simulink model "slidemodecontrol2"  (R2017b)
settings: Solver=ode45  StartTime=0.0  StopTime=2500  FixedStep=0.01  MaxStep=0.04  RelTol=1e-3
values from neighbouring files (symbols this model uses):
  azi0 = 90/180*pi    (= 1.57079632679)    [MonteCarlo_f.m]    (also in MonteCarlo_l.m; MonteCarlo_s.m; calcu_delta.m = 0.174532925199; calcu_delta11.m)
  cd0 = 0.024    [flight_sim.m]
  cd1 = 7.24e-4    (= 0.000724)    [flight_sim.m]
  cd2 = 0.406    [flight_sim.m]
  cl0 = -0.2317    [flight_sim.m]
  cl1 = 0.0513    [flight_sim.m]
  cl2 = 0.2945    [flight_sim.m]
  delta_d = delta_d0(ii)    [MonteCarlo_f.m]    (also in MonteCarlo_l.m; MonteCarlo_s.m; calcu_delta11.m = -0.08; calcu_delta3.m = -0.079)
  delta_l = delta_l0(ii)    [MonteCarlo_f.m]    (also in MonteCarlo_l.m; MonteCarlo_s.m; calcu_delta3.m = 0.05)
  fpa0 = theta_0(ii)    [MonteCarlo_f.m]    (also in MonteCarlo_l.m; MonteCarlo_s.m; calcu_delta.m = -0.0349065850399; calcu_delta11.m = -0.0349065850399)
  hs = 7320    [constant.m]    (also in flight_sim.m)
  lat0 = 0    [MonteCarlo_f.m]    (also in MonteCarlo_l.m; MonteCarlo_s.m; calcu_delta.m; calcu_delta11.m)
  lon0 = 0    [MonteCarlo_f.m]    (also in MonteCarlo_l.m; MonteCarlo_s.m; calcu_delta.m; calcu_delta11.m)
  m = 92079.25    [constant.m]    (also in flight_sim.m = 907.2)
  r0 = r_0(ii)    [MonteCarlo_f.m]    (also in MonteCarlo_l.m; MonteCarlo_s.m; calcu_delta.m = Re+97500; calcu_delta11.m = Re+100000)
  Re = 6371393    [calcu_R.m]    (also in calcu_R2.m; calcu_c.m; constant.m = 6378145; flight_sim.m)
  rho0 = rho_0(ii)    [MonteCarlo_f.m]    (also in MonteCarlo_l.m; MonteCarlo_s.m; constant.m = 1.225; flight_sim.m = 1.225)
  S = 249.9    [constant.m]    (also in flight_sim.m = 0.484)
  solution = output.result.solution    [calcu_A_B.m]    (also in calcu_A_B1.m; calcu_A_B2.m; main_bank.m)
  V0 = V_0(ii)    [MonteCarlo_f.m]    (also in MonteCarlo_l.m; MonteCarlo_s.m; calcu_delta.m = 7900; calcu_delta11.m = 7900)
undefined symbols (not defined in the file or in its folder): mu
settings Model: NumberOfSteps=500  Creator=ztyab  LastModifiedBy=ztyab
settings DataIOCC: SaveFormat=Array

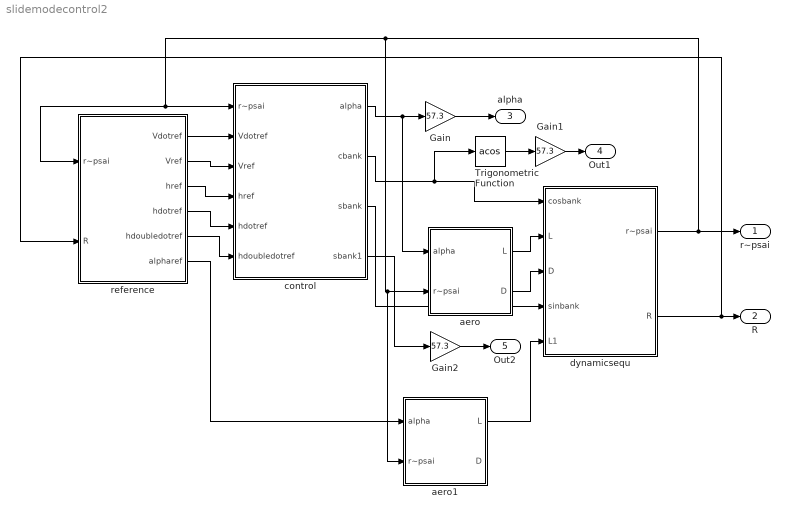
== system slidemodecontrol2 ==
  Gain : Gain  Gain=57.3
  Gain1 : Gain  Gain=57.3
  Gain2 : Gain  Gain=57.3
  Trigonometric Function : Trigonometry  Operator=acos
  aero : Subsystem
  aero1 : Subsystem
  control : Subsystem
  dynamicsequ : Subsystem
  reference : Subsystem
  r~psai : Outport
  R : Outport  Port=2
  alpha : Outport  Port=3
  Out1 : Outport  Port=4
  Out2 : Outport  Port=5
  wires:
  aero/1(L) -> dynamicsequ/2(L)
  dynamicsequ/1(r~psai) -> control/1(r~psai), reference/1(r~psai), aero1/2(r~psai), aero/2(r~psai), r~psai/1
  dynamicsequ/2(R) -> reference/2(R), R/1
  control/1(alpha) -> aero/1(alpha), Gain/1
  aero/2(D) -> dynamicsequ/3(D)
  control/2(cbank) -> Trigonometric Function/1, dynamicsequ/1(cosbank)
  control/3(sbank) -> dynamicsequ/4(sinbank)
  reference/1(Vdotref) -> control/2(Vdotref)
  reference/2(Vref) -> control/3(Vref)
  reference/3(href) -> control/4(href)
  reference/4(hdotref) -> control/5(hdotref)
  reference/5(hdoubledotref) -> control/6(hdoubledotref)
  Gain/1 -> alpha/1
  Trigonometric Function/1 -> Gain1/1
  Gain1/1 -> Out1/1
  control/4(sbank1) -> Gain2/1
  Gain2/1 -> Out2/1
  reference/6(alpharef) -> aero1/1(alpha)
  aero1/1(L) -> dynamicsequ/5(L1)

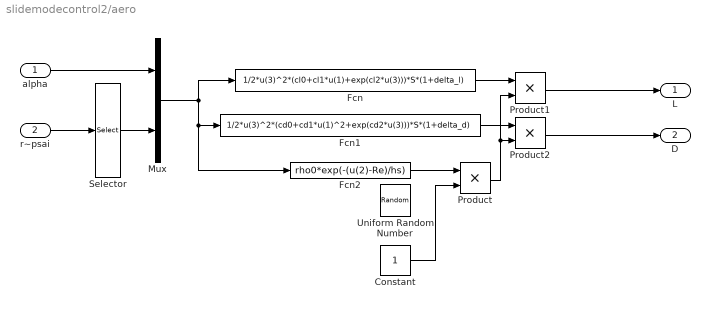
== system slidemodecontrol2/aero ==
  alpha : Inport
  r~psai : Inport  Port=2
  Constant : Constant
  Fcn : Fcn  Expr=1/2*u(3)^2*(cl0+cl1*u(1)+exp(cl2*u(3)))*S*(1+delta_l)
  Fcn1 : Fcn  Expr=1/2*u(3)^2*(cd0+cd1*u(1)^2+exp(cd2*u(3)))*S*(1+delta_d)
  Fcn2 : Fcn  Expr=rho0*exp(-(u(2)-Re)/hs)
  Mux : Mux  Inputs=2
  Product : Product
  Product1 : Product
  Product2 : Product
  Selector : Selector  InputPortWidth=6  IndexOptions=Index vector (dialog)  Indices=[1 4]  OutputSizes=1
  Uniform Random Number : UniformRandomNumber  Minimum=0.5  Maximum=1.5  SampleTime=0.01
  L : Outport
  D : Outport  Port=2
  wires:
  Mux/1 -> Fcn1/1, Fcn2/1, Fcn/1
  alpha/1 -> Mux/1
  r~psai/1 -> Selector/1
  Selector/1 -> Mux/2
  Fcn2/1 -> Product/1
  Product/1 -> Product1/2, Product2/2
  Fcn/1 -> Product1/1
  Fcn1/1 -> Product2/1
  Product1/1 -> L/1
  Product2/1 -> D/1
  Constant/1 -> Product/2

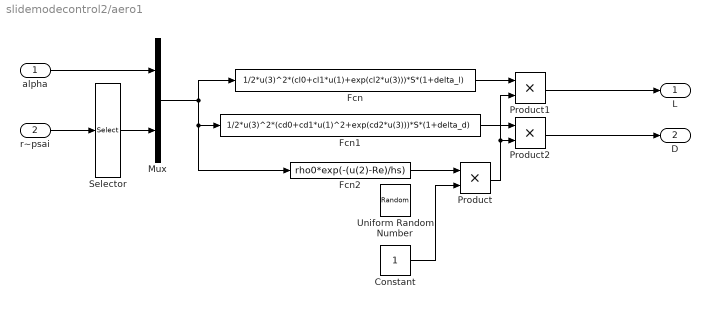
== system slidemodecontrol2/aero1 ==
  alpha : Inport
  r~psai : Inport  Port=2
  Constant : Constant
  Fcn : Fcn  Expr=1/2*u(3)^2*(cl0+cl1*u(1)+exp(cl2*u(3)))*S*(1+delta_l)
  Fcn1 : Fcn  Expr=1/2*u(3)^2*(cd0+cd1*u(1)^2+exp(cd2*u(3)))*S*(1+delta_d)
  Fcn2 : Fcn  Expr=rho0*exp(-(u(2)-Re)/hs)
  Mux : Mux  Inputs=2
  Product : Product
  Product1 : Product
  Product2 : Product
  Selector : Selector  InputPortWidth=6  IndexOptions=Index vector (dialog)  Indices=[1 4]  OutputSizes=1
  Uniform Random Number : UniformRandomNumber  Minimum=0.5  Maximum=1.5  SampleTime=0.01
  L : Outport
  D : Outport  Port=2
  wires:
  Mux/1 -> Fcn1/1, Fcn2/1, Fcn/1
  alpha/1 -> Mux/1
  r~psai/1 -> Selector/1
  Selector/1 -> Mux/2
  Fcn2/1 -> Product/1
  Product/1 -> Product1/2, Product2/2
  Fcn/1 -> Product1/1
  Fcn1/1 -> Product2/1
  Product1/1 -> L/1
  Product2/1 -> D/1
  Constant/1 -> Product/2

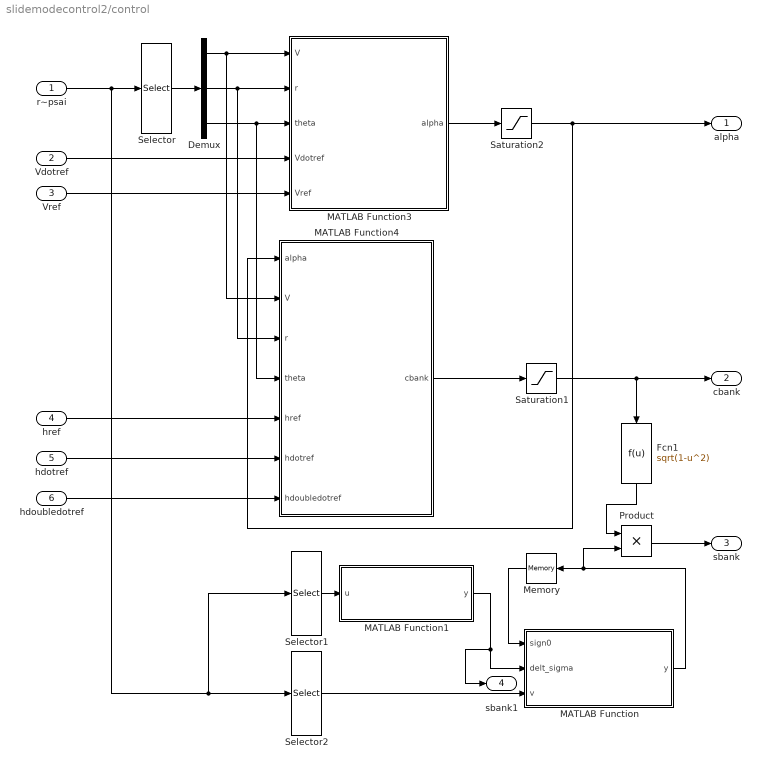
== system slidemodecontrol2/control ==
  r~psai : Inport
  Vdotref : Inport  Port=2
  Vref : Inport  Port=3
  href : Inport  Port=4
  hdotref : Inport  Port=5
  hdoubledotref : Inport  Port=6
  Demux : Demux  Outputs=3
  Fcn1 : Fcn  Expr=sqrt(1-u^2)
  MATLAB Function : MATLAB Function  TreatAsAtomicUnit=on
  MATLAB Function1 : MATLAB Function  TreatAsAtomicUnit=on
  MATLAB Function3 : MATLAB Function  TreatAsAtomicUnit=on
  MATLAB Function4 : MATLAB Function  TreatAsAtomicUnit=on
  Memory : Memory
  Product : Product
  Saturation1 : Saturate  UpperLimit=1  LowerLimit=cos(88/180*pi)
  Saturation2 : Saturate  UpperLimit=24*pi/180  LowerLimit=6*pi/180
  Selector : Selector  InputPortWidth=6  IndexOptions=Index vector (dialog)  Indices=[4 1 5]  OutputSizes=1
  Selector1 : Selector  InputPortWidth=6  IndexOptions=Index vector (dialog)  Indices=[2 3 6]  OutputSizes=1
  Selector2 : Selector  InputPortWidth=6  IndexOptions=Index vector (dialog)  Indices=[4]  OutputSizes=1
  alpha : Outport
  cbank : Outport  Port=2
  sbank : Outport  Port=3
  sbank1 : Outport  Port=4
  wires:
  Memory/1 -> MATLAB Function/1(sign0)
  Selector2/1 -> MATLAB Function/3(v)
  r~psai/1 -> Selector2/1, Selector1/1, Selector/1
  MATLAB Function/1(y) -> Product/2, Memory/1
  Product/1 -> sbank/1
  Selector1/1 -> MATLAB Function1/1(u)
  Selector/1 -> Demux/1
  href/1 -> MATLAB Function4/5(href)
  Fcn1/1 -> Product/1
  MATLAB Function4/1(cbank) -> Saturation1/1
  Saturation1/1 -> cbank/1, Fcn1/1
  Demux/2 -> MATLAB Function3/2(r), MATLAB Function4/3(r)
  Demux/1 -> MATLAB Function3/1(V), MATLAB Function4/2(V)
  Demux/3 -> MATLAB Function3/3(theta), MATLAB Function4/4(theta)
  Saturation2/1 -> MATLAB Function4/1(alpha), alpha/1
  hdotref/1 -> MATLAB Function4/6(hdotref)
  hdoubledotref/1 -> MATLAB Function4/7(hdoubledotref)
  MATLAB Function1/1(y) -> sbank1/1, MATLAB Function/2(delt_sigma)
  Vref/1 -> MATLAB Function3/5(Vref)
  Vdotref/1 -> MATLAB Function3/4(Vdotref)
  MATLAB Function3/1(alpha) -> Saturation2/1

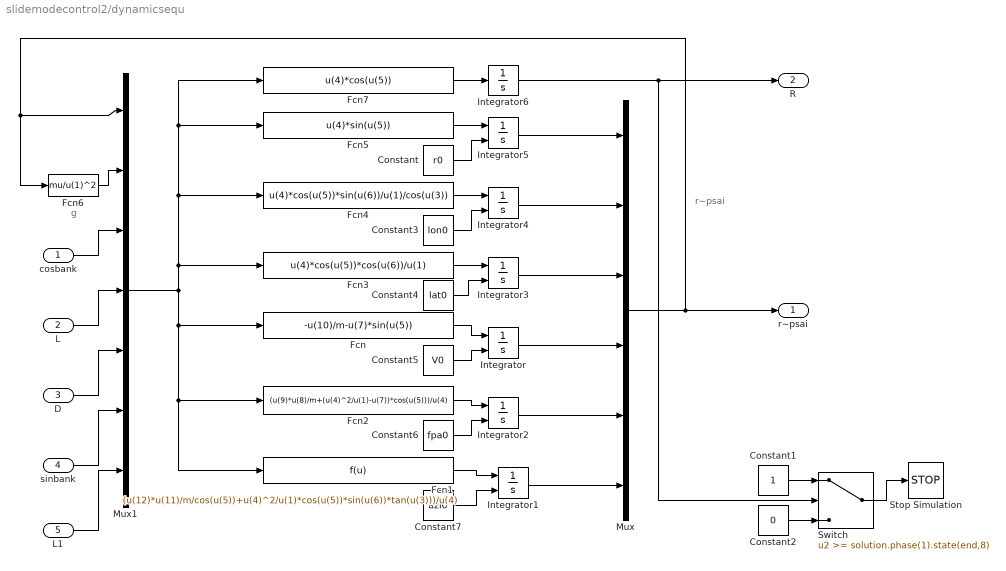
== system slidemodecontrol2/dynamicsequ ==
  note: g
  note: r~psai
  cosbank : Inport
  L : Inport  Port=2
  D : Inport  Port=3
  sinbank : Inport  Port=4
  L1 : Inport  Port=5
  Constant : Constant  Value=r0
  Constant1 : Constant
  Constant2 : Constant  Value=0
  Constant3 : Constant  Value=lon0
  Constant4 : Constant  Value=lat0
  Constant5 : Constant  Value=V0
  Constant6 : Constant  Value=fpa0
  Constant7 : Constant  Value=azi0
  Fcn : Fcn  Expr=-u(10)/m-u(7)*sin(u(5))
  Fcn1 : Fcn  Expr=(u(12)*u(11)/m/cos(u(5))+u(4)^2/u(1)*cos(u(5))*sin(u(6))*tan(u(3)))/u(4)
  Fcn2 : Fcn  Expr=(u(9)*u(8)/m+(u(4)^2/u(1)-u(7))*cos(u(5)))/u(4)
  Fcn3 : Fcn  Expr=u(4)*cos(u(5))*cos(u(6))/u(1)
  Fcn4 : Fcn  Expr=u(4)*cos(u(5))*sin(u(6))/u(1)/cos(u(3))
  Fcn5 : Fcn  Expr=u(4)*sin(u(5))
  Fcn6 : Fcn  Expr=mu/u(1)^2
  Fcn7 : Fcn  Expr=u(4)*cos(u(5))
  Integrator : Integrator  InitialConditionSource=external  InitialCondition=7500
  Integrator1 : Integrator  InitialConditionSource=external  InitialCondition=10*pi/180
  Integrator2 : Integrator  InitialConditionSource=external  InitialCondition=-2/180*pi
  Integrator3 : Integrator  InitialConditionSource=external
  Integrator4 : Integrator  InitialConditionSource=external
  Integrator5 : Integrator  InitialConditionSource=external  InitialCondition=95000+6371393
  Integrator6 : Integrator
  Mux : Mux  Inputs=6
  Mux1 : Mux  Inputs=7
  Stop Simulation : Stop
  Switch : Switch  Threshold=solution.phase(1).state(end,8)
  r~psai : Outport
  R : Outport  Port=2
  wires:
  Fcn6/1 -> Mux1/2
  Mux/1 -> Fcn6/1, Mux1/1, r~psai/1
  Fcn1/1 -> Integrator1/1
  Integrator1/1 -> Mux/6
  Fcn2/1 -> Integrator2/1
  Integrator4/1 -> Mux/2
  Fcn/1 -> Integrator/1
  Integrator2/1 -> Mux/5
  Fcn4/1 -> Integrator4/1
  Integrator3/1 -> Mux/3
  Fcn3/1 -> Integrator3/1
  Integrator/1 -> Mux/4
  Fcn5/1 -> Integrator5/1
  Integrator5/1 -> Mux/1
  L/1 -> Mux1/4
  D/1 -> Mux1/5
  cosbank/1 -> Mux1/3
  Mux1/1 -> Fcn1/1, Fcn2/1, Fcn/1, Fcn4/1, Fcn7/1, Fcn5/1, Fcn3/1
  Fcn7/1 -> Integrator6/1
  Integrator6/1 -> Switch/2, R/1
  Constant2/1 -> Switch/3
  Constant1/1 -> Switch/1
  Switch/1 -> Stop Simulation/1
  Constant/1 -> Integrator5/2
  Constant3/1 -> Integrator4/2
  Constant4/1 -> Integrator3/2
  Constant5/1 -> Integrator/2
  Constant6/1 -> Integrator2/2
  Constant7/1 -> Integrator1/2
  sinbank/1 -> Mux1/6
  L1/1 -> Mux1/7

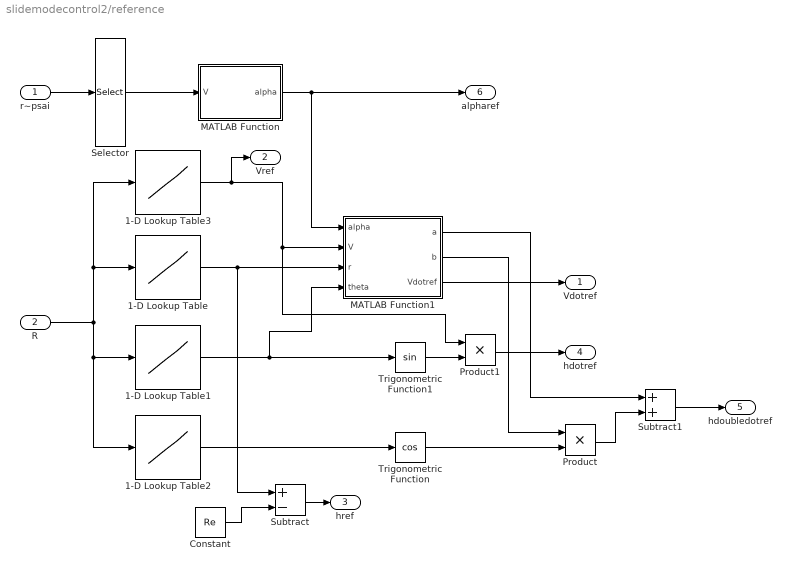
== system slidemodecontrol2/reference ==
  r~psai : Inport
  R : Inport  Port=2
  1-D Lookup Table : Lookup_n-D  NumberOfTableDimensions=1  BreakpointsForDimension1=solution.phase(1).state(:,8)  Table=solution.phase(1).state(:,1)  InterpMethod=Cubic spline  ExtrapMethod=Cubic spline  InternalRulePriority=Speed  RndMeth=Simplest  InputSameDT=on
  1-D Lookup Table1 : Lookup_n-D  NumberOfTableDimensions=1  BreakpointsForDimension1=solution.phase(1).state(:,8)  Table=solution.phase(1).state(:,5)  InterpMethod=Cubic spline  ExtrapMethod=Cubic spline  InternalRulePriority=Speed  RndMeth=Simplest  InputSameDT=on
  1-D Lookup Table2 : Lookup_n-D  NumberOfTableDimensions=1  BreakpointsForDimension1=solution.phase(1).state(:,8)  Table=solution.phase(1).state(:,7)  InterpMethod=Cubic spline  ExtrapMethod=Cubic spline  InternalRulePriority=Speed  RndMeth=Simplest  InputSameDT=on
  1-D Lookup Table3 : Lookup_n-D  NumberOfTableDimensions=1  BreakpointsForDimension1=solution.phase(1).state(:,8)  Table=solution.phase(1).state(:,4)  InterpMethod=Cubic spline  ExtrapMethod=Cubic spline  InternalRulePriority=Speed  RndMeth=Simplest  InputSameDT=on
  Constant : Constant  Value=Re
  MATLAB Function : MATLAB Function  TreatAsAtomicUnit=on
  MATLAB Function1 : MATLAB Function  TreatAsAtomicUnit=on
  Product : Product
  Product1 : Product
  Selector : Selector  InputPortWidth=6  IndexOptions=Index vector (dialog)  Indices=[4]  OutputSizes=1
  Subtract : Sum  Inputs=+-
  Subtract1 : Sum
  Trigonometric Function : Trigonometry  Operator=cos
  Trigonometric Function1 : Trigonometry
  Vdotref : Outport
  Vref : Outport  Port=2
  href : Outport  Port=3
  hdotref : Outport  Port=4
  hdoubledotref : Outport  Port=5
  alpharef : Outport  Port=6
  wires:
  1-D Lookup Table2/1 -> Trigonometric Function/1
  Trigonometric Function/1 -> Product/2
  Product1/1 -> hdotref/1
  R/1 -> 1-D Lookup Table2/1, 1-D Lookup Table1/1, 1-D Lookup Table3/1, 1-D Lookup Table/1
  MATLAB Function/1(alpha) -> alpharef/1, MATLAB Function1/1(alpha)
  Product/1 -> Subtract1/2
  Subtract1/1 -> hdoubledotref/1
  MATLAB Function1/2(b) -> Product/1
  Trigonometric Function1/1 -> Product1/2
  MATLAB Function1/1(a) -> Subtract1/1
  1-D Lookup Table1/1 -> MATLAB Function1/4(theta), Trigonometric Function1/1
  Selector/1 -> MATLAB Function/1(V)
  r~psai/1 -> Selector/1
  1-D Lookup Table/1 -> Subtract/1, MATLAB Function1/3(r)
  1-D Lookup Table3/1 -> Vref/1, MATLAB Function1/2(V), Product1/1
  MATLAB Function1/3(Vdotref) -> Vdotref/1
  Subtract/1 -> href/1
  Constant/1 -> Subtract/2

== matlab function slidemodecontrol2/control/MATLAB Function1 ==
  data: u input; y output
function y = fcn(u)
lambda=u(1);
phi=u(2);
sigma=u(3);
lambdaf=48*pi/180;
phif=60*pi/180;
if phi>phif
    sigma_t=pi-asin(cos(phif)*sin(lambdaf-lambda)/sin(acos(sin(phif)*sin(phi)+cos(phif)*cos(phi)*cos(lambdaf-lambda))));
else
    sigma_t=asin(cos(phif)*sin(lambdaf-lambda)/sin(acos(sin(phif)*sin(phi)+cos(phif)*cos(phi)*cos(lambdaf-lambda))));
end
y=sigma-sigma_t;
end

== matlab function slidemodecontrol2/reference/MATLAB Function ==
  data: V input; alpha output
function alpha = calcu_alpha(V)

v1=6500;
v2=5000;
alpha0=20*pi/180;
alphaf=10*pi/180;
alpha=(alpha0.*(V>v1)+((V-v1)*(alphaf-alpha0)/(v2-v1)+alpha0).*(V<=v1&V>=v2)+alphaf.*(V<v2));

end

== matlab function slidemodecontrol2/control/MATLAB Function ==
  data: sign0 input; y output; delt_sigma input; v input
function y = fcn(sign0,delt_sigma,v)

%#codegen
delt_sigma1=10/180*pi;
delt_sigma2=20/180*pi;
delt_sigma3=5/180*pi;
if (v>=6000)
    if (delt_sigma>delt_sigma1)
        sign=-1;
    elseif (delt_sigma<=delt_sigma1)&&(delt_sigma>=-delt_sigma1)
        sign=sign0;
    else 
        sign=1;
    end
elseif (4000<=v&v<6000)
    if (delt_sigma>delt_sigma2)
        sign=-1;
    elseif (delt_sigma<=delt_sigma2)&&(delt_sigma>=-delt_sigma2)
        sign=sign0;
    else 
        sign=1;
    end
elseif (3000<=v&&v<4000)
    delt=delt_sigma3+(delt_sigma2-delt_sigma3)/(4000-3000)*(v-3000);
    if (delt_sigma>delt)
        sign=-1;
    elseif (delt_sigma<=delt)&&(delt_sigma>=-delt)
        sign=sign0;
    else 
        sign=1;
    end  
else
    if (delt_sigma>delt_sigma3)
        sign=-1;
    elseif (delt_sigma<=delt_sigma3)&&(delt_sigma>=-delt_sigma3)
        sign=sign0;
    else 
        sign=1;
    end  
end
if(sign0==0)
    sign=1;
end
y =sign;
end

== matlab function slidemodecontrol2/reference/MATLAB Function1 ==
  data: alpha input; a output; V input; r input; theta input; b output; Vdotref output
function [a,b,Vdotref] = fcn(alpha,V,r,theta)
m=498.95;
S=0.113;
cd2 = -0.05119/340;
cd1 = 0.001944*57.3^2;
cd0 = -0.03795;
cl2 = 0.0017/340;
cl1 = 0.07412*57.3;
cl0 = -0.998;
rho0=1.225;
g0=9.81;
Re=6371393;
mu=g0*Re^2;
hs=7320;
Cl=exp(cl2*V)+cl1*alpha+cl0;
Cd=exp(cd2*V)+cd1*alpha.^2+cd0;
rho=rho0.*exp(-(r-Re)./hs);
q=1/2*rho.*V.^2;
L=q.*Cl.*S;
D=q.*Cd.*S;
g=mu./r.^2;

a=-D/m*sin(theta)-g+V^2*cos(theta)^2/r;
b=L*cos(theta)/m;
Vdotref=-D/m-g*sin(theta);

end

== matlab function slidemodecontrol2/control/MATLAB Function3 ==
  data: V input; r input; theta input; alpha output; Vdotref input; Vref input
function alpha = fcn(V,r,theta,Vdotref,Vref)
beta=1.3;
eta=2;
phi1=0.1*V;

m=498.95;
S=0.113;
rho0=1.225;
g0=9.81;
Re=6371393;
mu=g0*Re^2;
hs=7320;
rho=rho0.*exp(-(r-Re)./hs);
q=1/2*rho.*V.^2;
g=mu./r.^2;

b_1=-q*S/m;
f_1=-g*sin(theta);

k_1=beta*eta+(beta-1)*abs(f_1-Vdotref);
s=V-Vref;
if(abs(s/phi1)<=1)
    sat=s/phi1;
else
    sat=sign(s/phi1);
end
u=abs(1/b_1*(Vdotref-f_1-k_1*sat));

sdot=f_1+b_1*u-Vdotref;
kkk=sdot*s+eta*abs(s);
cd2 = -0.05119/340;
cd1 = 0.001944*57.3^2;
cd0 = -0.03795;

if u-exp(cd2*V)-cd0<=0
    alpha1=10/180*pi;
else
    alpha1=sqrt((u-exp(cd2*V)-cd0)/cd1);
end
alpha=alpha1;
% f=@(x)exp(cd2*V)+cd1*x.^2+cd0-u;
% alpha=fzero(f,15/180*pi);
end

== matlab function slidemodecontrol2/control/MATLAB Function4 ==
  data: alpha input; V input; r input; theta input; cbank output; href input; hdotref input; hdoubledotref input
function cbank = fcn(alpha,V,r,theta,href,hdotref,hdoubledotref)
beta=1.3;
eta=500;
phi=0.05*href;
lambda=100;
F_f=0.3;

m=498.95;
S=0.113;
rho0=1.225;
g0=9.81;
Re=6371393;
mu=g0*Re^2;
hs=7320;
rho=rho0.*exp(-(r-Re)./hs);
q=1/2*rho.*V.^2;
g=mu./r.^2;
cd2 = -0.05119/340;
cd1 = 0.001944*57.3^2;
cd0 = -0.03795;
cl2 = 0.0017/340;
cl1 = 0.07412*57.3;
cl0 = -0.998;
Cl=exp(cl2*V)+cl1*alpha+cl0;
Cd=exp(cd2*V)+cd1*alpha.^2+cd0;
L=q.*Cl.*S;
D=q.*Cd.*S;

b_2=L/m*cos(theta);
f_2=-g-D/m*sin(theta)+V^2*(cos(theta))^2/r;
hdot=V*sin(theta);

F=abs(-D/m*F_f*sin(theta));
% F=F_f;

k_2=beta*(eta+F)+(beta-1)*abs(hdoubledotref-f_2-lambda*(hdot-hdotref));
s=hdot-hdotref+lambda*(r-Re-href);

if(abs(s/phi)<=1)
    sat=s/phi;
else
    sat=sign(s/phi);
end
cbank=1/b_2*(hdoubledotref-f_2-lambda*(hdot-hdotref)-k_2*sat);
hdoubledot=f_2+b_2*cbank;
sdot=hdoubledot-hdoubledotref+lambda*(hdot-hdotref);
kkk=s*sdot+eta*abs(s);
end
